simulink model "rct_suspension"  (R2022a)
settings: Solver=ode23t  StartTime=0.0  StopTime=2  MaxStep=0.2  RelTol=1e-3  EnableMultiTasking=on
model workspace (MATLAB code in the model file):
  | Mb = 300; % Body mass (kg)
  | Mw = 60;  % Wheel assembly mass (kg)
  | Bs = 1000;   % Shock absorber between car body and wheel assembly (N/m/s)
  | Ks = 16000 ; % Spring between car body and wheel assembly (N/m)
  | Kt = 190000; % Compressibility of the pneumatic tire(N/m)
  | Ta = 60; % Actuator parameter
libraries: fl_lib x13, nesl_utility x8, simulink_extras x1
settings Model: Creator=The MathWorks, Inc.  LastModifiedBy=The MathWorks, Inc.
settings SolverCC: AlgebraicLoopSolver=TrustRegion  MaxZcPerStep=1
settings DataIOCC: LimitDataPoints=on  SaveFormat=Array  ReturnWorkspaceOutputs=off
settings OptimizationCC: LifeSpan=inf
settings DebuggingCC: SolverPrmCheckMsg=warning  UnconnectedInputMsg=warning  UnconnectedOutputMsg=warning  UnconnectedLineMsg=warning  AllowSymbolicDim=off  SFUnexpectedBacktrackingDiag=warning  SFNoUnconditionalDefaultTransitionDiag=warning  SFExecutionAtInitializationDiag=none  SFMachineParentedDataDiag=warning  ArithmeticOperatorsInVariantConditions=warning
settings HardwareCC: ProdBitPerPointer=32  ProdBitPerSizeT=32  ProdBitPerPtrDiffT=32  ProdLargestAtomicFloat=None  ProdIntDivRoundTo=Undefined  ProdEndianess=Unspecified  ProdWordSize=32  ProdHWDeviceType=32-bit Generic
settings ModelReferenceCC: PropagateSignalLabelsOutOfModel=off
settings SFSimCC: SimUseLocalCustomCode=off  CustomCodeUndefinedFunction=UseInterfaceOnly
settings RTWCC: RTWUseLocalCustomCode=off  DLArmComputeVersion=19.05
settings CodeAppCC: StateflowObjectComments=on
settings GRTTargetCC: TargetLangStandard=C89/C90 (ANSI)
settings ConfigComp: CovMetricSettings=dw  CovSaveCumulativeToWorkspaceVar=on  CovSaveSingleToWorkspaceVar=on  CovExternalEMLEnable=off  CovSFcnEnable=off
settings SimscapeCC: SimscapeNormalizeSystem=off

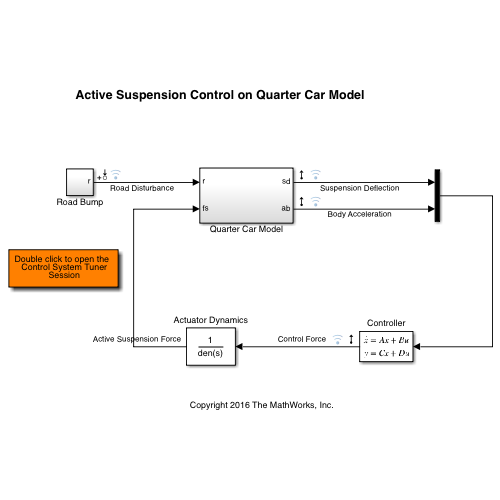
[thumbnail: Simulink's stored preview of the top-level diagram]
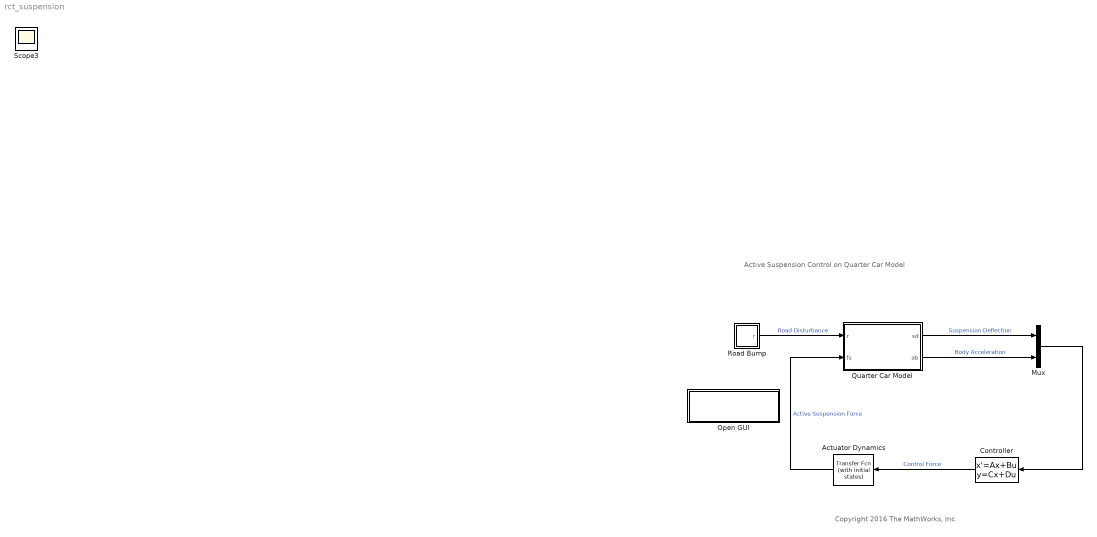
== system rct_suspension ==
  note: Copyright 2016 The MathWorks, Inc.
  note: Active Suspension Control on Quarter Car Model
  Actuator Dynamics : simulink_extras/Additional Linear/Transfer Fcn (with initial states)  N=[1]  D="[1/Ta  1]"  X0=0
  Controller : StateSpace  A=eye(2)  B=eye(2)  C=[0 0]  D=[0 0]  InitialCondition=0
  Mux : Mux  Inputs=2
  Open GUI : Subsystem
      settings: RTWMemSecFuncInitTerm=Default  RTWMemSecFuncExecute=Default  RTWMemSecDataConstants=Default  RTWMemSecDataInternal=Default  RTWMemSecDataParameters=Default
      settings: OpenFcn=|
      | Wroad = ss(0.07);
      | HandlingTarget = 0.044444 * tf([1/8 1],[1/80 1]);
      | ComfortTarget = 0.6667 * tf([1/0.45 1],[1/150 1]);
      | Wact = tf(0.1684*[1 500],[1 50]);
      | controlSystemTuner('SessionFileForActiveSuspensionQuarterCar');
      mask Display: disp('Double click to open the \n Control System Tuner\n Session')
  Quarter Car Model : Subsystem
  Road Bump : Subsystem
  Scope3 : Scope
  wires:
  Road Bump/1(r) -> Quarter Car Model/1(r)  "Road Disturbance"
  Actuator Dynamics/1 -> Quarter Car Model/2(fs)  "Active Suspension Force"
  Quarter Car Model/1(sd) -> Mux/1  "Suspension Deflection"
  Quarter Car Model/2(ab) -> Mux/2  "Body Acceleration"
  Controller/1 -> Actuator Dynamics/1  "Control Force"
  Mux/1 -> Controller/1

== system rct_suspension/Open GUI ==

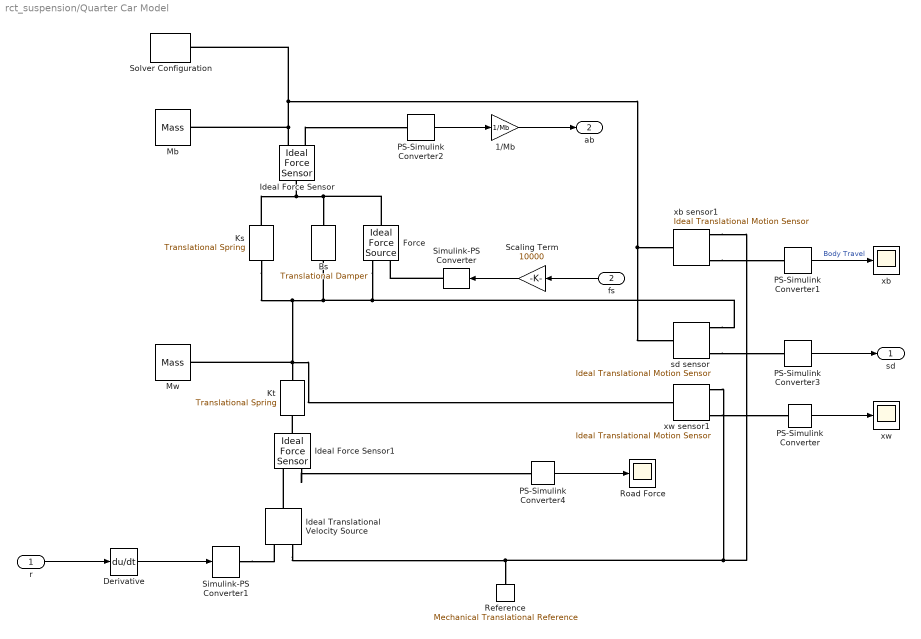
== system rct_suspension/Quarter Car Model ==
  r : Inport
  fs : Inport  Port=2
  1/Mb : Gain  Gain=1/Mb
  Bs : fl_lib/Mechanical/Translational Elements/Translational Damper  D=Bs N/(m/s)  v_specify=off  v_priority=High  v=0 m/s  v_nominal_specify=off  v_nominal_unit=m/s  v_nominal_value=1  f_specify=off  f_priority=High  f=0 N  f_nominal_specify=off  f_nominal_unit=N  f_nominal_value=1
      settings: SourceProductBaseCode=PW,SS,VE
  Derivative : Derivative  CoefficientInTFapproximation=1e-4
  Force : fl_lib/Mechanical/Mechanical Sources/Ideal Force Source
      settings: SourceProductBaseCode=PW,SS,VE
  Ideal Force Sensor : fl_lib/Mechanical/Mechanical Sensors/Ideal Force Sensor
      settings: SourceProductBaseCode=PW,SS,VE
  Ideal Force Sensor1 : fl_lib/Mechanical/Mechanical Sensors/Ideal Force Sensor
      settings: SourceProductBaseCode=PW,SS,VE
  Ideal Translational Velocity Source : fl_lib/Mechanical/Mechanical Sources/Ideal Translational Velocity Source
      settings: SourceProductBaseCode=PW,SS,VE
  Ks : fl_lib/Mechanical/Translational Elements/Translational Spring  spr_rate=Ks N/m  v_specify=off  v_priority=High  v=0 m/s  v_nominal_specify=off  v_nominal_unit=m/s  v_nominal_value=1  f_specify=off  f_priority=High  f=0 N  f_nominal_specify=off  f_nominal_unit=N  f_nominal_value=1  x_specify=off  x_priority=High  x=0 m  x_nominal_specify=off  x_nominal_unit=m  x_nominal_value=1
      settings: SourceProductBaseCode=PW,SS,VE
  Kt : fl_lib/Mechanical/Translational Elements/Translational Spring  spr_rate=Kt N/m  v_specify=off  v_priority=High  v=0 m/s  v_nominal_specify=off  v_nominal_unit=m/s  v_nominal_value=1  f_specify=off  f_priority=High  f=0 N  f_nominal_specify=off  f_nominal_unit=N  f_nominal_value=1  x_specify=off  x_priority=High  x=0 m  x_nominal_specify=off  x_nominal_unit=m  x_nominal_value=1
      settings: SourceProductBaseCode=PW,SS,VE
  Mb : fl_lib/Mechanical/Translational Elements/Mass  mass=Mb kg  num_ports=foundation.enum.numPorts2.one  v_specify=off  v_priority=High  v=0 m/s  v_nominal_specify=off  v_nominal_unit=m/s  v_nominal_value=1  f_specify=off  f_priority=High  f=0 N  f_nominal_specify=off  f_nominal_unit=N  f_nominal_value=1
      settings: SourceProductBaseCode=PW,SS,VE
  Mw : fl_lib/Mechanical/Translational Elements/Mass  mass=Mw kg  num_ports=foundation.enum.numPorts2.one  v_specify=off  v_priority=High  v=0 m/s  v_nominal_specify=off  v_nominal_unit=m/s  v_nominal_value=1  f_specify=off  f_priority=High  f=0 N  f_nominal_specify=off  f_nominal_unit=N  f_nominal_value=1
      settings: SourceProductBaseCode=PW,SS,VE
  PS-Simulink Converter{,1..4} (5 alike) : nesl_utility/PS-Simulink Converter  PhysicalDomain=network_engine_domain  SubClassName=ps_output  LeftPortType=input  RightPortType=output  PseudoPeriodic=off  Frequencies=[]  VectorFormat=1-D array  Unit=1  AffineConversion=off
      settings: SourceProductBaseCode=SS,PW,VE
  Reference : fl_lib/Mechanical/Translational Elements/Mechanical Translational Reference
      settings: SourceProductBaseCode=PW,SS,VE
  Road Force : Scope
  Scaling Term : Gain  Gain=10000
  Simulink-PS Converter : nesl_utility/Simulink-PS Converter  PhysicalDomain=network_engine_domain  SubClassName=ps_input  LeftPortType=input  RightPortType=output  PseudoPeriodic=off  Frequencies=[]  NoiseDistribution=none  NoiseParameters=[]  Unit=N  AffineConversion=off  FilteringAndDerivatives=zero  SimscapeFilterOrder=1  InputFilterTimeConstant=0.001  UdotUserProvided=1
      settings: SourceProductBaseCode=SS,PW,VE
  Simulink-PS Converter1 : nesl_utility/Simulink-PS Converter  PhysicalDomain=network_engine_domain  SubClassName=ps_input  LeftPortType=input  RightPortType=output  PseudoPeriodic=off  Frequencies=[]  NoiseDistribution=none  NoiseParameters=[]  Unit=1  AffineConversion=off  FilteringAndDerivatives=zero  SimscapeFilterOrder=1  InputFilterTimeConstant=0.001  UdotUserProvided=1
      settings: SourceProductBaseCode=SS,PW,VE
  Solver Configuration : nesl_utility/Solver Configuration  PhysicalDomain=network_engine_domain  SubClassName=solver  LeftPortType=input  RightPortType=generic  Tones=[]  Harmonics=[]  SimulateNoise=off  Profile=off  UseLocalSampling=off  EnableSwitchedLinearOptims=on  FrequencyDomain=off  UseCCode=off  RelTol=0.001  AbsTol=1e-06  MinStep=1e-09  ToWorkspace=off  RevertToSquareIcSolve=off  NumHomotopyIterations=100  PhasorMode=off  PhasorModeNumHarmonics=1  IndexReductionMethod=DerivativeReplacement  DoDC=off  ResidualTolerance=1e-09  UseLocalSolver=off  LocalSolverChoice=NE_BACKWARD_EULER_ADVANCER  LocalSolverSampleTime=0.001  DoFixedCost=off  MaxNonlinIter=3  MaxModeIter=2  ComputeImpulses=off  ImpulseIterations=2  LinearAlgebra=Sparse  LinearAlgebraNumThread=0  EquationFormulation=NE_TIME_EF  DelaysMemoryBudget=1024  AutomaticFiltering=on  FilteringTimeConstant=0.001  PartitionStorageMethod=AS_NEEDED  PartitionMemoryBudget=1024  PartitionMethod=FAST
      settings: SourceProductBaseCode=SS,PW,VE
  sd sensor : fl_lib/Mechanical/Mechanical Sensors/Ideal Translational Motion Sensor  offset=0 m
      settings: SourceProductBaseCode=PW,SS,VE
  xb : Scope
  xb sensor1 : fl_lib/Mechanical/Mechanical Sensors/Ideal Translational Motion Sensor  offset=0 m
      settings: SourceProductBaseCode=PW,SS,VE
  xw : Scope
  xw sensor1 : fl_lib/Mechanical/Mechanical Sensors/Ideal Translational Motion Sensor  offset=0 m
      settings: SourceProductBaseCode=PW,SS,VE
  sd : Outport
  ab : Outport  Port=2
  wires:
  fs/1 -> Scaling Term/1
  PS-Simulink Converter1/1 -> xb/1  "Body Travel"
  PS-Simulink Converter/1 -> xw/1
  PS-Simulink Converter3/1 -> sd/1
  1/Mb/1 -> ab/1
  Derivative/1 -> Simulink-PS Converter1/1
  PS-Simulink Converter4/1 -> Road Force/1
  PS-Simulink Converter2/1 -> 1/Mb/1
  r/1 -> Derivative/1
  Scaling Term/1 -> Simulink-PS Converter/1
  connections:
  xb sensor1/RConn3 -- PS-Simulink Converter1/LConn1
  Ks/RConn1 -- sd sensor/RConn1 -- Force/RConn2 -- Bs/RConn1 -- xw sensor1/LConn1 -- Mw/LConn1 -- Kt/LConn1
  xw sensor1/RConn3 -- PS-Simulink Converter/LConn1
  Ideal Force Sensor/RConn2 -- PS-Simulink Converter2/LConn1
  sd sensor/RConn3 -- PS-Simulink Converter3/LConn1
  Simulink-PS Converter1/RConn1 -- Ideal Translational Velocity Source/RConn1
  Ideal Translational Velocity Source/RConn2 -- xb sensor1/RConn1 -- xw sensor1/RConn1 -- Reference/LConn1
  Ideal Translational Velocity Source/LConn1 -- Ideal Force Sensor1/RConn1
  Ideal Force Sensor1/LConn1 -- Kt/RConn1
  Ideal Force Sensor1/RConn2 -- PS-Simulink Converter4/LConn1
  Ks/LConn1 -- Ideal Force Sensor/LConn1 -- Bs/LConn1 -- Force/LConn1
  Ideal Force Sensor/RConn1 -- xb sensor1/LConn1 -- sd sensor/LConn1 -- Solver Configuration/RConn1 -- Mb/LConn1
  Simulink-PS Converter/RConn1 -- Force/RConn1

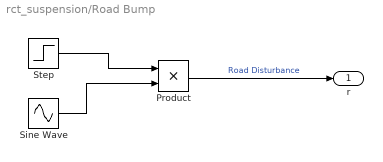
== system rct_suspension/Road Bump ==
  Product : Product
  Sine Wave : Sin  Amplitude=-0.025  Bias=0.025  Frequency=8*pi  Phase=pi/2  SampleTime=0
  Step : Step  Time=0.25  Before=1  After=0  SampleTime=0
  r : Outport
  wires:
  Sine Wave/1 -> Product/2
  Product/1 -> r/1  "Road Disturbance"
  Step/1 -> Product/1
